simulink model "constant_f_V"  (R2016a)
settings: Solver=FixedStepAuto  StartTime=0.0  StopTime=3  FixedStep=0.0001  RelTol=1e-3
undefined symbols (not defined in the file): Lm, Lr, Ls, M_abc2ab0, Rr, sig
settings Model: Creator=ebenera  LastModifiedBy=ebenera

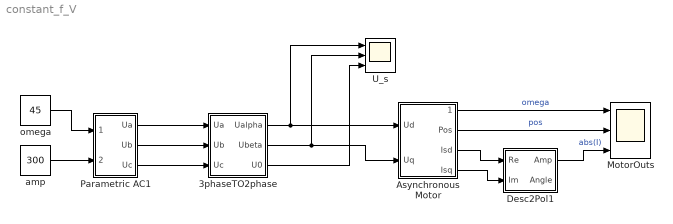
== system constant_f_V ==
  "3phaseTO2phase " : Subsystem
  Asynchronous Motor : Subsystem
  Desc2Pol1 : Subsystem
  MotorOuts : Scope  NumInputPorts=3
  Parametric AC1 : Subsystem
  U_s : Scope  NumInputPorts=3
  amp : Constant  Value=300
  omega : Constant  Value=45
  wires:
  "3phaseTO2phase "/1(Ualpha) -> U_s/1, Asynchronous Motor/1(Ud)
  "3phaseTO2phase "/2(Ubeta) -> Asynchronous Motor/2(Uq), U_s/2
  "3phaseTO2phase "/3(U0) -> U_s/3
  Asynchronous Motor/4(Isq) -> Desc2Pol1/2(Im)
  Asynchronous Motor/3(Isd) -> Desc2Pol1/1(Re)
  amp/1 -> Parametric AC1/2(Amp)
  Parametric AC1/1(Ua) -> "3phaseTO2phase "/1(Ua)
  Parametric AC1/2(Ub) -> "3phaseTO2phase "/2(Ub)
  Parametric AC1/3(Uc) -> "3phaseTO2phase "/3(Uc)
  omega/1 -> Parametric AC1/1(Omega)
  Desc2Pol1/1(Amp) -> MotorOuts/3  "abs(I)"
  Asynchronous Motor/1(Omega) -> MotorOuts/1  "omega"
  Asynchronous Motor/2(Pos) -> MotorOuts/2  "pos"

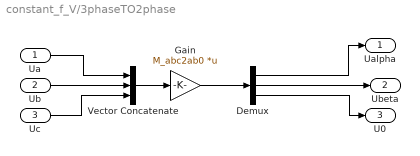
== system constant_f_V/3phaseTO2phase  ==
  Ua : Inport
  Ub : Inport  Port=2
  Uc : Inport  Port=3
  Demux : Demux  Outputs=3
  Gain : Gain  Gain=M_abc2ab0  Multiplication=Matrix(K*u)
  Vector Concatenate : Concatenate  NumInputs=3
  Ualpha : Outport
  Ubeta : Outport  Port=2
  U0 : Outport  Port=3
  wires:
  Vector Concatenate/1 -> Gain/1
  Ua/1 -> Vector Concatenate/1
  Demux/3 -> U0/1
  Gain/1 -> Demux/1
  Uc/1 -> Vector Concatenate/3
  Ub/1 -> Vector Concatenate/2
  Demux/1 -> Ualpha/1
  Demux/2 -> Ubeta/1

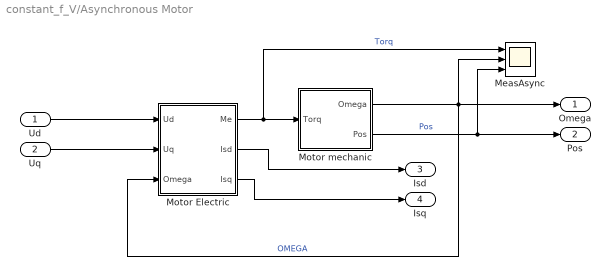
== system constant_f_V/Asynchronous Motor ==
  Ud : Inport
  Uq : Inport  Port=2
  MeasAsync : Scope  NumInputPorts=3
  Motor Electric : Subsystem
  Motor mechanic : Subsystem
  Omega : Outport
  Pos : Outport  Port=2
  Isd : Outport  Port=3
  Isq : Outport  Port=4
  wires:
  Motor mechanic/2(Pos) -> MeasAsync/3, Pos/1  "Pos"
  Motor mechanic/1(Omega) -> Motor Electric/3(Omega), Omega/1, MeasAsync/2  "OMEGA"
  Motor Electric/1(Me) -> MeasAsync/1, Motor mechanic/1("Torq ")  "Torq"
  Motor Electric/2(Isd) -> Isd/1
  Motor Electric/3(Isq) -> Isq/1
  Uq/1 -> Motor Electric/2(Uq)
  Ud/1 -> Motor Electric/1(Ud)

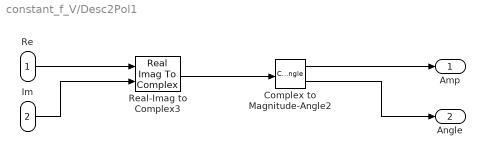
== system constant_f_V/Desc2Pol1 ==
  Re : Inport
  Im : Inport  Port=2
  Complex to Magnitude-Angle2 : ComplexToMagnitudeAngle
  Real-Imag to Complex3 : RealImagToComplex
  Amp : Outport
  Angle : Outport  Port=2
  wires:
  Complex to Magnitude-Angle2/1 -> Amp/1
  Real-Imag to Complex3/1 -> Complex to Magnitude-Angle2/1
  Complex to Magnitude-Angle2/2 -> Angle/1
  Re/1 -> Real-Imag to Complex3/1
  Im/1 -> Real-Imag to Complex3/2

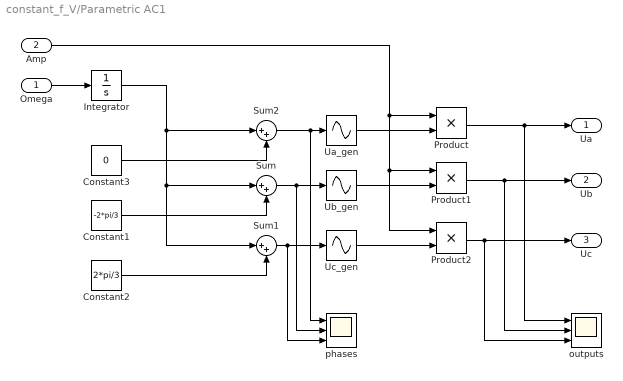
== system constant_f_V/Parametric AC1 ==
  Omega : Inport
  Amp : Inport  Port=2
  Constant1 : Constant  Value=-2*pi/3
  Constant2 : Constant  Value=2*pi/3
  Constant3 : Constant  Value=0
  Integrator : Integrator  WrapState=on
  Product : Product
  Product1 : Product
  Product2 : Product
  Sum : Sum  Inputs=|++
  Sum1 : Sum  Inputs=|++
  Sum2 : Sum  Inputs=|++
  Ua_gen : Sin  TimeSource=Use external signal  SampleTime=0
  Ub_gen : Sin  TimeSource=Use external signal  SampleTime=0
  Uc_gen : Sin  TimeSource=Use external signal  SampleTime=0
  outputs : Scope  NumInputPorts=3
  phases : Scope  NumInputPorts=3
  Ua : Outport
  Ub : Outport  Port=2
  Uc : Outport  Port=3
  wires:
  Sum/1 -> phases/2, Ub_gen/1
  Omega/1 -> Integrator/1
  Constant1/1 -> Sum/2
  Constant2/1 -> Sum1/2
  Sum1/1 -> phases/3, Uc_gen/1
  Sum2/1 -> phases/1, Ua_gen/1
  Constant3/1 -> Sum2/2
  Integrator/1 -> Sum2/1, Sum1/1, Sum/1
  Product/1 -> Ua/1, outputs/1
  Product2/1 -> outputs/3, Uc/1
  Product1/1 -> Ub/1, outputs/2
  Amp/1 -> Product/1, Product2/1, Product1/1
  Ua_gen/1 -> Product/2
  Uc_gen/1 -> Product2/2
  Ub_gen/1 -> Product1/2

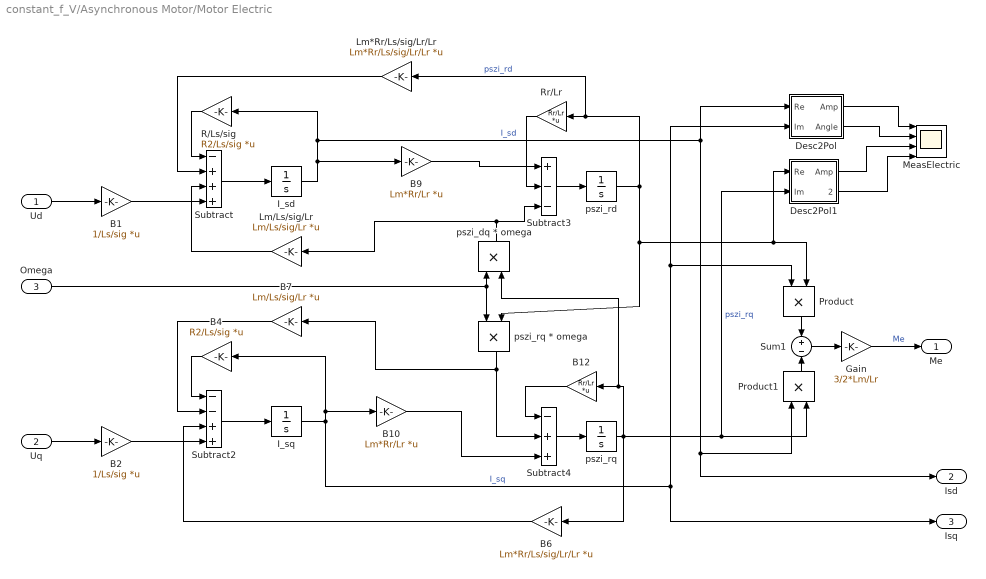
== system constant_f_V/Asynchronous Motor/Motor Electric ==
  Ud : Inport
  Uq : Inport  Port=2
  Omega : Inport  Port=3
  B1 : Gain  Gain=1/Ls/sig  Multiplication=Matrix(K*u)
  B10 : Gain  Gain=Lm*Rr/Lr  Multiplication=Matrix(K*u)
  B12 : Gain  Gain=Rr/Lr  Multiplication=Matrix(K*u)
  B2 : Gain  Gain=1/Ls/sig  Multiplication=Matrix(K*u)
  B4 : Gain  Gain=R2/Ls/sig  Multiplication=Matrix(K*u)
  B6 : Gain  Gain=Lm*Rr/Ls/sig/Lr/Lr  Multiplication=Matrix(K*u)
  B7 : Gain  Gain=Lm/Ls/sig/Lr  Multiplication=Matrix(K*u)
  B9 : Gain  Gain=Lm*Rr/Lr  Multiplication=Matrix(K*u)
  Desc2Pol : Subsystem
  Desc2Pol1 : Subsystem
  Gain : Gain  Gain=3/2*Lm/Lr
  I_sd : Integrator
  I_sq : Integrator
  Lm*Rr/Ls/sig/Lr/Lr : Gain  Gain=Lm*Rr/Ls/sig/Lr/Lr  Multiplication=Matrix(K*u)
  Lm/Ls/sig/Lr : Gain  Gain=Lm/Ls/sig/Lr  Multiplication=Matrix(K*u)
  MeasElectric : Scope  NumInputPorts=4
  Product : Product
  Product1 : Product
  R/Ls/sig : Gain  Gain=R2/Ls/sig  Multiplication=Matrix(K*u)
  Rr/Lr : Gain  Gain=Rr/Lr  Multiplication=Matrix(K*u)
  Subtract : Sum  Inputs=-+++
  Subtract2 : Sum  Inputs=--++
  Subtract3 : Sum  Inputs=+--
  Subtract4 : Sum  Inputs=-++
  Sum1 : Sum  Inputs=+-
  pszi_dq * omega : Product
  pszi_rd : Integrator
  "pszi_rq " : Integrator
  pszi_rq * omega : Product
  Me : Outport
  Isd : Outport  Port=2
  Isq : Outport  Port=3
  wires:
  pszi_rq * omega/1 -> Subtract4/2, B7/1
  Subtract/1 -> I_sd/1
  B12/1 -> Subtract4/1
  Product1/1 -> Sum1/2
  Lm*Rr/Ls/sig/Lr/Lr/1 -> Subtract/2
  Product/1 -> Sum1/1
  I_sq/1 -> Product/1, Desc2Pol/2(Im), Isq/1, B10/1, B4/1  "I_sq"
  I_sd/1 -> B9/1, Isd/1, Product1/1, Desc2Pol/1(Re), R/Ls/sig/1  "I_sd"
  Sum1/1 -> Gain/1
  R/Ls/sig/1 -> Subtract/1
  B6/1 -> Subtract2/3
  B4/1 -> Subtract2/1
  pszi_dq * omega/1 -> Subtract3/3, Lm/Ls/sig/Lr/1
  Omega/1 -> pszi_rq * omega/1, pszi_dq * omega/1
  B9/1 -> Subtract3/1
  Rr/Lr/1 -> Subtract3/2
  pszi_rd/1 -> Product/2, Desc2Pol1/1(Re), pszi_rq * omega/2, Lm*Rr/Ls/sig/Lr/Lr/1, Rr/Lr/1  "pszi_rd"
  Lm/Ls/sig/Lr/1 -> Subtract/3
  "pszi_rq "/1 -> B6/1, Product1/2, Desc2Pol1/2(Im), pszi_dq * omega/2, B12/1  "pszi_rq"
  B7/1 -> Subtract2/2
  Gain/1 -> Me/1  "Me"
  B10/1 -> Subtract4/3
  Subtract4/1 -> "pszi_rq "/1
  Subtract2/1 -> I_sq/1
  Subtract3/1 -> pszi_rd/1
  Uq/1 -> B2/1
  Ud/1 -> B1/1
  B1/1 -> Subtract/4
  B2/1 -> Subtract2/4
  Desc2Pol/1(Amp) -> MeasElectric/1
  Desc2Pol/2(Angle) -> MeasElectric/2
  Desc2Pol1/1(Amp) -> MeasElectric/3
  Desc2Pol1/2(Angle) -> MeasElectric/4

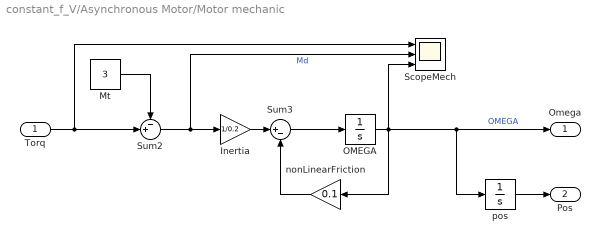
== system constant_f_V/Asynchronous Motor/Motor mechanic ==
  "Torq " : Inport
  Inertia : Gain  Gain=1/0.2
  Mt : Constant  Value=3
  OMEGA : Integrator
  ScopeMech : Scope  NumInputPorts=3
  Sum2 : Sum  Inputs=-+|
  Sum3 : Sum  Inputs=|+-
  nonLinearFriction : Gain  Gain=0.1
  pos : Integrator  WrapState=on
  Omega : Outport
  Pos : Outport  Port=2
  wires:
  "Torq "/1 -> ScopeMech/1, Sum2/2
  OMEGA/1 -> ScopeMech/3, pos/1, Omega/1, nonLinearFriction/1  "OMEGA"
  Sum3/1 -> OMEGA/1
  Sum2/1 -> Inertia/1, ScopeMech/2  "Md"
  Mt/1 -> Sum2/1
  nonLinearFriction/1 -> Sum3/2
  Inertia/1 -> Sum3/1
  pos/1 -> Pos/1

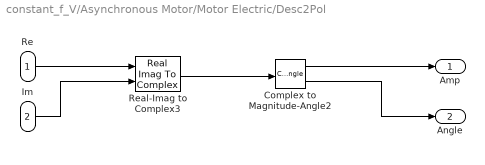
== system constant_f_V/Asynchronous Motor/Motor Electric/Desc2Pol ==
  Re : Inport
  Im : Inport  Port=2
  Complex to Magnitude-Angle2 : ComplexToMagnitudeAngle
  Real-Imag to Complex3 : RealImagToComplex
  Amp : Outport
  Angle : Outport  Port=2
  wires:
  Complex to Magnitude-Angle2/1 -> Amp/1
  Real-Imag to Complex3/1 -> Complex to Magnitude-Angle2/1
  Complex to Magnitude-Angle2/2 -> Angle/1
  Re/1 -> Real-Imag to Complex3/1
  Im/1 -> Real-Imag to Complex3/2

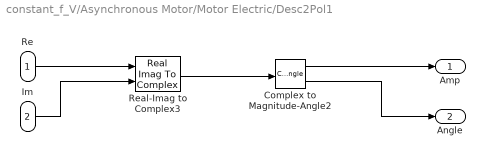
== system constant_f_V/Asynchronous Motor/Motor Electric/Desc2Pol1 ==
  Re : Inport
  Im : Inport  Port=2
  Complex to Magnitude-Angle2 : ComplexToMagnitudeAngle
  Real-Imag to Complex3 : RealImagToComplex
  Amp : Outport
  Angle : Outport  Port=2
  wires:
  Complex to Magnitude-Angle2/1 -> Amp/1
  Real-Imag to Complex3/1 -> Complex to Magnitude-Angle2/1
  Complex to Magnitude-Angle2/2 -> Angle/1
  Re/1 -> Real-Imag to Complex3/1
  Im/1 -> Real-Imag to Complex3/2
